simulink model "agg_all_simulated_unitIDs_example"  (R2015a)
settings: Solver=ode3  StartTime=0.0  StopTime=10.0  FixedStep=1  RelTol=1e-3
libraries: libAggregators x1, libSimulators x1
settings Model: Creator=jcardena  LastModifiedBy=jcardena

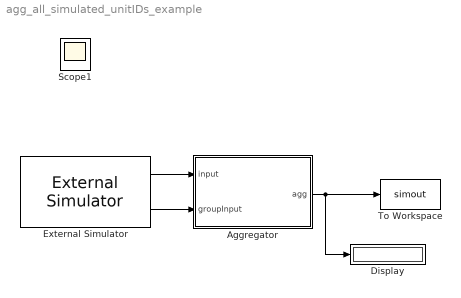
== system agg_all_simulated_unitIDs_example ==
  Aggregator : Subsystem  BlockChoice=Simplest
      settings: AttributesFormatString=%<BlockChoice>  TemplateBlock=libAggregators/Aggregator  MemberBlocks=Average,Simple,Simple db Aggregator,Simplest
  Display : Display
  External Simulator : libSimulators/External Simulator  Condition=%20151211%  N=10  db_name=HeatingUnits  db_username=sw_ETS  db_password=unb.sql.2015
  To Workspace : ToWorkspace  VariableName=simout  SaveFormat=Structure With Time  SampleTime=-1
  Scope1 : Scope
  wires:
  External Simulator/2 -> Aggregator/2(groupInput)
  External Simulator/1 -> Aggregator/1(input)
  Aggregator/1(agg) -> Display/1, To Workspace/1

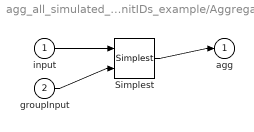
== system agg_all_simulated_unitIDs_example/Aggregator ==
  input : Inport
  groupInput : Inport  Port=2
  Simplest : libAggregators/Simplest  SystemSampleTime=-1
  agg : Outport
  wires:
  input/1 -> Simplest/1
  groupInput/1 -> Simplest/2
  Simplest/1 -> agg/1
